simulink model "SupervisorStateMachine"  (Simulink 8.9)
settings: Solver=FixedStepDiscrete  StartTime=0.0  StopTime=10.0  RelTol=1e-3
settings Model: Creator=yuchao  LastModifiedBy=jonkro
settings DataIOCC: LimitDataPoints=off  SaveFormat=Structure  SignalLoggingSaveFormat=Dataset
settings OptimizationCC: UseDivisionForNetSlopeComputation=on  LifeSpan=auto
settings DebuggingCC: UnderspecifiedInitializationDetection=Simplified  MergeDetectMultiDrivingBlocksExec=error  FcnCallInpInsideContextMsg=error  StateNameClashWarn=none  SFUnexpectedBacktrackingDiag=error  SFNoUnconditionalDefaultTransitionDiag=error  SFExecutionAtInitializationDiag=warning
settings HardwareCC: ProdBitPerLong=64  ProdBitPerPointer=64  ProdBitPerSizeT=64  ProdBitPerPtrDiffT=64  ProdLargestAtomicFloat=Float  ProdIntDivRoundTo=Zero  ProdEndianess=LittleEndian  ProdWordSize=64  ProdHWDeviceType=Intel->x86-64 (Linux 64)
settings ModelReferenceCC: PropagateSignalLabelsOutOfModel=on
settings RTWCC: GenCodeOnly=on  PackageGeneratedCodeAndArtifacts=on  PackageName=SupervisorCodez  GenerateReport=on  Toolchain=Microsoft Windows SDK v7.1 | nmake (64-bit Windows)  LaunchReport=on  TargetLang=C++
settings GRTTargetCC: TargetLangStandard=C++03 (ISO)  GeneratePreprocessorConditionals=Use local settings  CombineOutputUpdateFcns=on  MatFileLogging=off  MultiInstanceERTCode=on  CodeInterfacePackaging=C++ class  GRTInterface=off
settings CPPComponent: GenerateDestructor=on  GenerateExternalIOAccessMethods=None  ParameterMemberVisibility=private  InternalMemberVisibility=private  GenerateParameterAccessMethods=None  GenerateInternalMemberAccessMethods=None  UseOperatorNewForModelRefRegistration=off
settings ConfigComp: CovMetricSettings=dwe  CovHtmlReporting=off  CovSaveCumulativeToWorkspaceVar=off  CovSaveSingleToWorkspaceVar=off  CovExternalEMLEnable=on

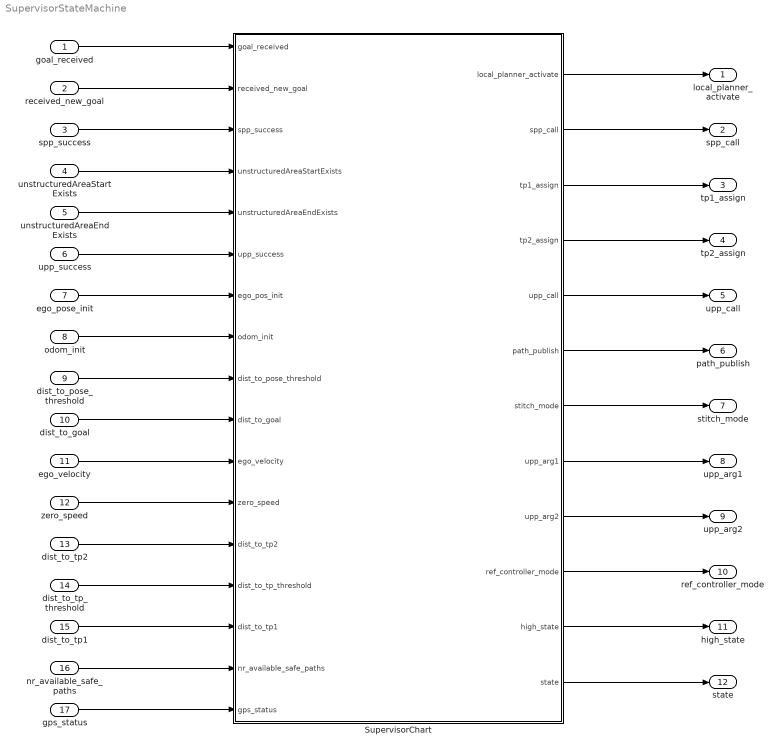
== system SupervisorStateMachine ==
  goal_received : Inport  OutDataTypeStr=boolean
  received_new_goal : Inport  Port=2  OutDataTypeStr=boolean
  spp_success : Inport  Port=3  OutDataTypeStr=boolean
  unstructuredAreaStartExists : Inport  Port=4  OutDataTypeStr=boolean
  unstructuredAreaEndExists : Inport  Port=5  OutDataTypeStr=boolean
  upp_success : Inport  Port=6  OutDataTypeStr=boolean
  ego_pose_init : Inport  Port=7  OutDataTypeStr=boolean
  odom_init : Inport  Port=8  OutDataTypeStr=boolean
  dist_to_pose_threshold : Inport  Port=9  OutDataTypeStr=double
  dist_to_goal : Inport  Port=10  OutDataTypeStr=double
  ego_velocity : Inport  Port=11  OutDataTypeStr=double
  zero_speed : Inport  Port=12  OutDataTypeStr=double
  dist_to_tp2 : Inport  Port=13  OutDataTypeStr=double
  dist_to_tp_threshold : Inport  Port=14  OutDataTypeStr=double
  dist_to_tp1 : Inport  Port=15  OutDataTypeStr=double
  nr_available_safe_paths : Inport  Port=16  OutDataTypeStr=int8
  gps_status : Inport  Port=17  OutDataTypeStr=uint8
  SupervisorChart : Stateflow chart  TreatAsAtomicUnit=on
  local_planner_activate : Outport  OutDataTypeStr=boolean
  spp_call : Outport  Port=2  OutDataTypeStr=boolean
  tp1_assign : Outport  Port=3  OutDataTypeStr=boolean
  tp2_assign : Outport  Port=4  OutDataTypeStr=boolean
  upp_call : Outport  Port=5  OutDataTypeStr=boolean
  path_publish : Outport  Port=6  OutDataTypeStr=boolean
  stitch_mode : Outport  Port=7  OutDataTypeStr=Enum: stitch_mode_dt
  upp_arg1 : Outport  Port=8  OutDataTypeStr=Enum: upp_arg_dt
  upp_arg2 : Outport  Port=9  OutDataTypeStr=Enum: upp_arg_dt
  ref_controller_mode : Outport  Port=10  OutDataTypeStr=Enum: ref_controller_mode_dt
  high_state : Outport  Port=11  OutDataTypeStr=Enum: high_state_dt
  state : Outport  Port=12  OutDataTypeStr=Enum: state_dt
  wires:
  goal_received/1 -> SupervisorChart/1(goal_received)
  received_new_goal/1 -> SupervisorChart/2(received_new_goal)
  spp_success/1 -> SupervisorChart/3(spp_success)
  unstructuredAreaStartExists/1 -> SupervisorChart/4(unstructuredAreaStartExists)
  unstructuredAreaEndExists/1 -> SupervisorChart/5(unstructuredAreaEndExists)
  upp_success/1 -> SupervisorChart/6(upp_success)
  ego_pose_init/1 -> SupervisorChart/7(ego_pos_init)
  odom_init/1 -> SupervisorChart/8(odom_init)
  dist_to_pose_threshold/1 -> SupervisorChart/9(dist_to_pose_threshold)
  dist_to_goal/1 -> SupervisorChart/10(dist_to_goal)
  ego_velocity/1 -> SupervisorChart/11(ego_velocity)
  zero_speed/1 -> SupervisorChart/12(zero_speed)
  dist_to_tp2/1 -> SupervisorChart/13(dist_to_tp2)
  dist_to_tp_threshold/1 -> SupervisorChart/14(dist_to_tp_threshold)
  dist_to_tp1/1 -> SupervisorChart/15(dist_to_tp1)
  SupervisorChart/1(local_planner_activate) -> local_planner_activate/1
  SupervisorChart/2(spp_call) -> spp_call/1
  SupervisorChart/3(tp1_assign) -> tp1_assign/1
  SupervisorChart/4(tp2_assign) -> tp2_assign/1
  SupervisorChart/5(upp_call) -> upp_call/1
  SupervisorChart/6(path_publish) -> path_publish/1
  SupervisorChart/7(stitch_mode) -> stitch_mode/1
  SupervisorChart/8(upp_arg1) -> upp_arg1/1
  SupervisorChart/9(upp_arg2) -> upp_arg2/1
  SupervisorChart/10(ref_controller_mode) -> ref_controller_mode/1
  nr_available_safe_paths/1 -> SupervisorChart/16(nr_available_safe_paths)
  SupervisorChart/11(high_state) -> high_state/1
  SupervisorChart/12(state) -> state/1
  gps_status/1 -> SupervisorChart/17(gps_status)

== stateflow chart SupervisorChart ==
  state Init
    en:
    path_publish = false;
    high_state = high_state_dt.state_init;
    spp_call = false;
    tp1_assign = false;
    tp2_assign = false;
    upp_call = false;
    stitch_mode = stitch_mode_dt.stitch_mode_unknown;
    upp_arg1 = upp_arg_dt.upp_arg_unknown;
    upp_arg2 = upp_arg_dt.upp_arg_unknown;
    ref_controller_mode = ref_controller_mode_dt.nominal;
    tp1_init = false;
    tp2_init = false;
    state WaitingForGoal
      % Waiting for the first goal message
      en:
      state = state_dt.state_waiting_for_goal;
    state Failed
      en:
      state = state_dt.state_failed;
    state Goal
      % Send stationary command
      en:
      state = state_dt.state_goal;
    state ParkingToRoad
      % Initialize tp1. Call UPP
      en:
      tp1_init = true;
      tp1_assign = true;
      upp_call = true;
      upp_arg1 = upp_arg_dt.ego_pose_arg;
      upp_arg2 = upp_arg_dt.tp1_pose_arg;
      state = state_dt.state_parking_to_road;
      ex:
      tp1_assign = false;
      upp_call = false;
    state ParkingToParking
      % Initialize tp1 and tp2. Call UPP
      en:
      tp1_init = true;
      tp2_init = true;
      tp1_assign = true;
      tp2_assign = true;
      upp_call = true;
      upp_arg1 = upp_arg_dt.ego_pose_arg;
      upp_arg2 = upp_arg_dt.tp1_pose_arg;
      state = state_dt.state_parking_to_parking;
      ex:
      tp1_assign = false;
      tp2_assign = false;
      upp_call = false;
    state CallForPlan
      % Activate the local planner and ask SPP to plan to the goal pose
      en:
      spp_call = true;
      local_planner_activate = true;
      state = state_dt.state_call_for_plan;
      ex:
      spp_call = false;
      local_planner_activate = false;
    state WaitForTransforms
      % Waiting for the ego pose and odometry transformations to be set up
      en:
      state = state_dt.state_wait_for_transforms;
    (junction 27) -> Failed [order 2] : [~upp_success]
    ParkingToParking -> (junction 27)
    ParkingToRoad -> (junction 27)
    (junction 28) -> ParkingToParking [order 1] : [unstructuredAreaEndExists]
    (junction 29) -> (junction 28) [order 1] : [unstructuredAreaStartExists]
    (junction 28) -> ParkingToRoad [order 2] : [~unstructuredAreaEndExists]
    Failed -> (junction 30)
    CallForPlan -> Failed [order 1] : [~spp_success]
    CallForPlan -> (junction 29) [order 2] : [spp_success]
    (junction 29) -> (junction 31) [order 2] : [~unstructuredAreaStartExists]
    WaitForTransforms -> CallForPlan : [odom_init && ego_pos_init]
    (junction 30) -> CallForPlan : [received_new_goal]
    (default) -> WaitingForGoal
    Goal -> (junction 30)
    WaitingForGoal -> WaitForTransforms : [goal_received]
  state FailureState
    en:
    high_state = high_state_dt.state_failure;
    state SafeStop
      en:
      state = state_dt.state_safe_stop;
    state EmergencyStop
      en:
      state = state_dt.state_emergency_stop;
    state AEB
      en:
      ref_controller_mode ...
      = ref_controller_mode_dt.emergency_maneuver;
      state = state_dt.state_aeb;
    state SSMP
      en:
      ref_controller_mode ...
      = ref_controller_mode_dt.safe_maneuver;
      state = state_dt.state_ssmp;
    (junction 47) -> SSMP [order 1] : [nr_available_safe_paths > 0]
    (junction 47) -> AEB [order 2] : [nr_available_safe_paths <= 0]
    SSMP -> SafeStop : [ego_velocity < zero_speed]
    AEB -> EmergencyStop : [ego_velocity < zero_speed]
  state Driving
    en:
    path_publish = true;
    ref_controller_mode...
    = ref_controller_mode_dt.nominal;
    high_state = high_state_dt.state_driving;
    state GoToGoal
      % Change stitch mode
      en:
      stitch_mode = stitch_mode_dt.upp;
      state = state_dt.state_go_to_goal;
    state WaitToLeaveTp2
      en:
      state = state_dt.state_wait_to_leave_tp2;
    state SPP
      % Change stitch mode
      en:
      stitch_mode = stitch_mode_dt.spp;
      state = state_dt.state_spp;
    state CloseToTransition2
      % Call UPP
      en:
      upp_call = true;
      upp_arg1 = upp_arg_dt.tp2_pose_arg;
      upp_arg2 = upp_arg_dt.goal_pose_arg;
      state = state_dt.state_close_to_tp2;
      ex:
      upp_call = false;
    state TransitionToSPP
      % Change stitch mode
      en:
      stitch_mode = stitch_mode_dt.upp_to_spp;
      state = state_dt.state_transition_to_spp;
    state WaitToLeaveTp1
      en:
      state = state_dt.state_wait_to_leave_tp1;
    state TransitionToUPP2
      % Change stitch mode.
      en:
      stitch_mode = stitch_mode_dt.spp_to_upp;
      state = state_dt.state_transition_to_upp2;
    state RoadToParking
      % Initialize tp2. Set stitch mode. Activate reference path.
      en:
      tp2_init = true;
      tp2_assign = true;
      path_publish = true;
      stitch_mode = stitch_mode_dt.spp;
      state = state_dt.state_road_to_parking;
      ex:
      tp2_assign = false;
    state RoadToRoad
      % Good to go! Set stitch mode. Activate reference path.
      en:
      path_publish = true;
      stitch_mode = stitch_mode_dt.spp;
      state = state_dt.state_road_to_road;
    state FromParking
      % Set stitch mode. Activate reference path.
      en:
      path_publish = true;
      stitch_mode = stitch_mode_dt.upp;
      state = state_dt.state_from_parking;
    FromParking -> TransitionToSPP : [dist_to_tp1 < dist_to_tp_threshold]
    TransitionToSPP -> WaitToLeaveTp1 : [dist_to_tp1 < dist_to_pose_threshold]
    WaitToLeaveTp1 -> (junction 53) : [dist_to_tp1 > dist_to_tp_threshold]
    RoadToParking -> (junction 52)
    SPP -> (junction 52)
    (junction 52) -> CloseToTransition2 : [dist_to_tp2 < dist_to_tp_threshold]
    (junction 53) -> SPP [order 2] : [tp2_init]
    (junction 53) -> RoadToRoad [order 1] : [~tp2_init]
    CloseToTransition2 -> TransitionToUPP2 [order 2] : [upp_success]
    RoadToRoad -> (junction 54)
    GoToGoal -> (junction 54)
    TransitionToUPP2 -> WaitToLeaveTp2 : [dist_to_tp2 < dist_to_pose_threshold]
    WaitToLeaveTp2 -> GoToGoal : [dist_to_tp2 > dist_to_tp_threshold]
  (default) -> Init
  Driving -> (junction 47) [order 1] : [gps_status ~= 1]
  (junction 27) -> FromParking [order 1] : [upp_success]
  CloseToTransition2 -> (junction 47) [order 1] : [~upp_success]
  (junction 31) -> RoadToParking [order 1] : [unstructuredAreaEndExists]
  (junction 100) -> (junction 30)
  (junction 31) -> RoadToRoad [order 2] : [~unstructuredAreaEndExists]
  EmergencyStop -> (junction 99)
  SafeStop -> (junction 99)
  (junction 54) -> Goal : [dist_to_goal < dist_to_pose_threshold && ego_velocity < zero_speed]
  (junction 99) -> (junction 100)
  Driving -> (junction 100) [order 2]
  data: goal_received input boolean; received_new_goal input boolean; spp_success input boolean; unstructuredAreaStartExists input boolean; unstructuredAreaEndExists input boolean; tp1_init local boolean =false; tp2_init local boolean =false; upp_success input boolean; ego_pos_init input boolean; odom_init input boolean; dist_to_pose_threshold input double; dist_to_goal input double; ego_velocity input double; zero_speed input double; dist_to_tp2 input double; dist_to_tp_threshold input double; dist_to_tp1 input double; local_planner_activate output boolean =false; spp_call output boolean =false; tp1_assign output boolean =false; tp2_assign output boolean =false; upp_call output boolean =false; path_publish output boolean =false; stitch_mode output Enum: stitch_mode_dt =stitch_mode_dt.stitch_mode_unknown; upp_arg1 output Enum: upp_arg_dt =upp_arg_dt.upp_arg_unknown; upp_arg2 output Enum: upp_arg_dt =upp_arg_dt.upp_arg_unknown; nr_available_safe_paths input int8; ref_controller_mode output Enum: ref_controller_mode_dt =ref_controller_mode_dt.ref_controller_mode_unknown; high_state output Enum: high_state_dt =high_state_dt.state_high_unknown; state output Enum: state_dt =state_dt.state_unknown; gps_status input uint8
